simulink model "paper_implementation_Aahana"  (R2024b)
settings: Solver=VariableStepAuto  StartTime=0.0  StopTime=inf  RelTol=1e-3
libraries: commsdrhw_v2 x1, dspsrcs4 x1
settings Model: Creator=ETE  LastModifiedBy=ETE

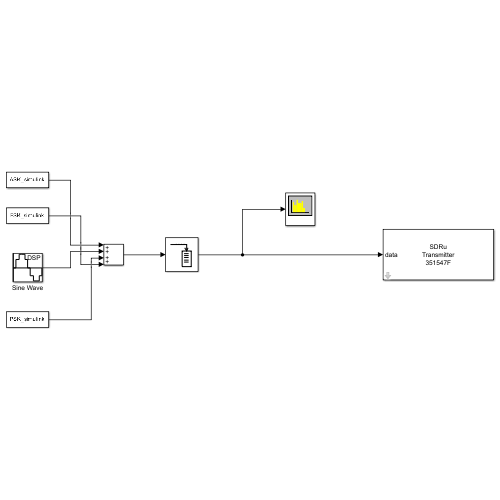
[thumbnail: Simulink's stored preview of the top-level diagram]
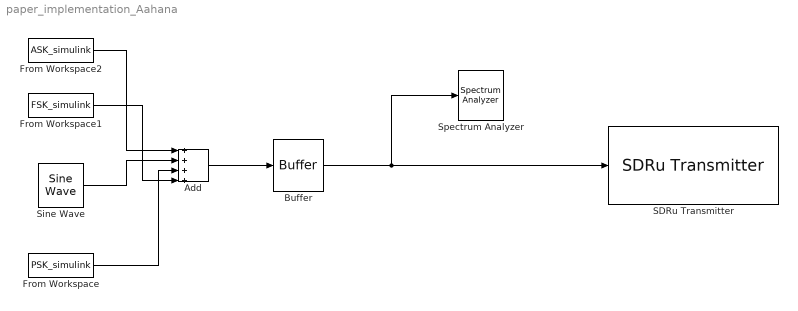
== system paper_implementation_Aahana ==
  Add : Sum  Inputs=++++
  Buffer : Buffer  OutputFrames=off
  From Workspace : FromWorkspace  VariableName=PSK_simulink  OutDataTypeStr=double  SampleTime=5e-7
  From Workspace1 : FromWorkspace  VariableName=FSK_simulink  OutDataTypeStr=double  SampleTime=5e-7
  From Workspace2 : FromWorkspace  VariableName=ASK_simulink  OutDataTypeStr=double  SampleTime=5e-7
  SDRu Transmitter : commsdrhw_v2/SDRu Transmitter  rxtx=tx  initializeIPAddress=0  devMap=0  USRP2_IP=192.168.10.2  USRP_IP_X300=192.168.10.2  USRP_IP_X310=192.168.10.2  USRP_IP_N300=No devices found  USRP_IP_N310=192.168.10.2  USRP_IP_N320=No devices found  USRP_serialNumB200=3136D21  USRP_serialNumB210=351547F  platform=B210  prevPlatform=B210  lastIPAddressPopup=192.168.10.2  USRP_ID=351547F  LastIPAddress=192.168.10.2  ChannelMapping=1  centerFrequencySrc=Dialog  centerFrequency=2.45e9  loOffsetSrc=Dialog  loOffset=1e6  gainSrc=Dialog  gain=32  PPSSource=Internal  clockSource=Internal  EnableGPSLock=off  EnsureSyncGPSTime=off  EnableTimeTrigger=off  triggerTime=5  enableMIMOCableSync=off  EnableRefLock=off  masterClkRateParam=10000000  masterClkRateB200=32e6  masterClkRateB210=10e6  masterClkRateX300=200e6  masterClkRateX310=200e6  masterClkRateN300=125e6  masterClkRateN310=125e6  masterClkRateN320=200e6  decimInterpSrc=Dialog  lastDecimSource=Dialog  decimInterp=5  USRP2_IP_NUM=[51 53 49 53 52 55 70]  frameLength=362  sampleRate=2000000  TransportDataType=int16  outputDatatype=Same as transport data type  overrunUnderrunPort=off  sampleTime=5.12e-06  dboardInfo=|  HOST_DATA_PORT=30000  HOST_CONTROL_PORT=30001  USRP2_DATA_PORT=32769  USRP2_CONTROL_PORT=32768  bufferMode=Continuous streaming  EnableBurstMode=off  NumFramesInBurst=100
      | dbid: 0
      |           dbName: 'no db found'
      |          freqMin: 0
      |          freqMax: 0
      |          gainMin: 0
      |          gainMax: 0
      |     gainStepSize: 0
  Sine Wave : dspsrcs4/Sine Wave  Amplitude=1  Frequency=100  Phase=0  SampleMode=Discrete  OutComplex=Complex  CompMethod=Trigonometric fcn  TableSize=Speed  SampleTime=0.000001  SamplesPerFrame=1024  ResetState=Restart at time zero  OutputFrames=off  dataType=single  wordLen=16  udDataType=sfix(16)  fracBitsMode=Best precision  numFracBits=15  OutDataTypeStr=single  LastOutDataTypeStr=single
  Spectrum Analyzer : SpectrumAnalyzer  WindowPosition=[749.000000,224.000000,800.000000,500.000000,]  Visible=on  ScopeFrameLocation=window  SampleRateSource=Property  SampleRate=2000000  PlotAsTwoSidedSpectrum=off  WindowInvariantSamplesPerUpdate=on  FrequencySpan=Start and stop frequencies  StartFrequency=0  StopFrequency=1000  YLimits=[-73.88840315860097,45.763181599699]  SelectedToolstripTab=spectrumAnalyzerToolstrip.measurementsTab
  wires:
  Buffer/1 -> SDRu Transmitter/1, Spectrum Analyzer/1
  Add/1 -> Buffer/1
  From Workspace2/1 -> Add/1
  From Workspace1/1 -> Add/4
  Sine Wave/1 -> Add/2
  From Workspace/1 -> Add/3
